simulink library "rpi_blkst"  (Simulink 7.6)
settings: Solver=ode45  StartTime=0.0  StopTime=10.0  RelTol=1e-3
settings Model: Creator=jacques  LastModifiedBy=jacques

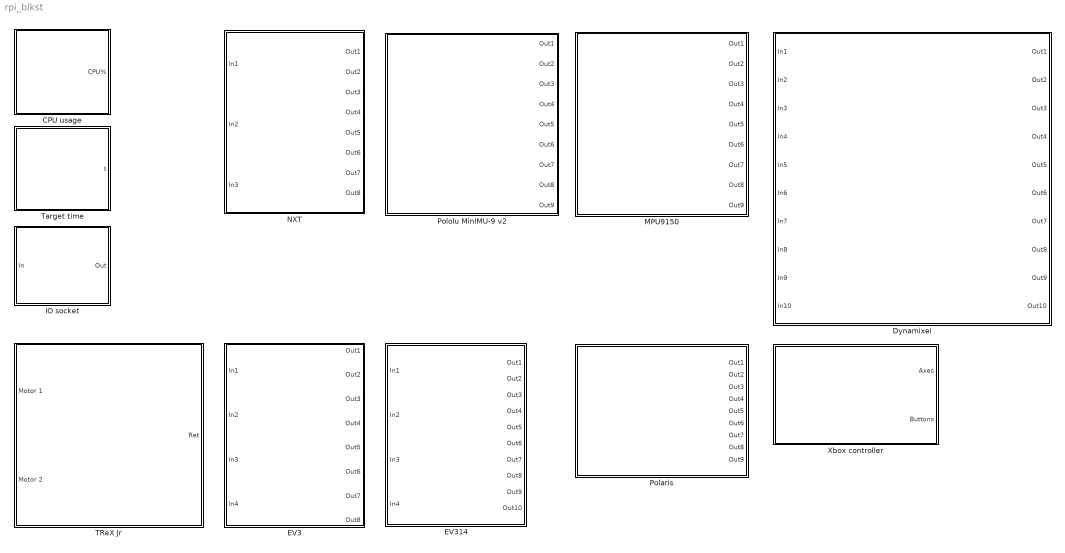
== system rpi_blkst ==
  CPU usage : Subsystem  mask(Target CPU usage){rpi_mask_Ts=0.01}
      mask prompts: rpi_mask_Ts "Sampling interval (s)"
      mask help: Percentage of CPU usage on the target. To be safe, keep below 80%.
      mask Help: Time spent in the system computation with respect to the period duration.
      mask Display: image(imread('cpu_usage.jpg'))
  Dynamixel : Subsystem  mask(Dynamixel actuator){rpi_mask_Ts=0.005, rpi_mask_portname=0, rpi_mask_baudrate=1000000, rpi_mask_startid=1, rpi_mask_nbid=1, rpi_mask_proto=2, rpi_mask_write_addr=0, rpi_mask_write_length=0, rpi_mask_read_addr=0, rpi_mask_read_length=0, rpi_mask_read_sign=0, rpi_mask_init1_addr=0, rpi_mask_init1_length=0, rpi_mask_init1_data=0, rpi_mask_init2_addr=0, rpi_mask_init2_length=0, rpi_mask_init2_data=0, rpi_mask_init3_addr=0, rpi_mask_init3_length=0, rpi_mask_init3_data=0, rpi_mask_init4_addr=0, rpi_mask_init4_length=0, rpi_mask_init4_data=0, rpi_mask_init5_addr=0, rpi_mask_init5_length=0, rpi_mask_init5_data=0, rpi_mask_init6_addr=0, rpi_mask_init6_length=0, rpi_mask_init6_data=0, rpi_mask_init7_addr=0, rpi_mask_init7_length=0, rpi_mask_init7_data=0, rpi_mask_init8_addr=0, rpi_mask_init8_length=0, rpi_mask_init8_data=0, rpi_mask_halt1_addr=0, rpi_mask_halt1_length=0, rpi_mask_halt1_data=0, rpi_mask_halt2_addr=0, rpi_mask_halt2_length=0, rpi_mask_halt2_data=0}
      mask prompts: rpi_mask_Ts "Sampling interval (s)"; rpi_mask_portname "Serial port number"; rpi_mask_baudrate "Baud rate (bps)"; rpi_mask_startid "ID of the first device"; rpi_mask_nbid "Number of devices"; rpi_mask_proto "Protocol version"; rpi_mask_write_addr "Input write address"; rpi_mask_write_length "Input write length"; rpi_mask_read_addr "Output read address"; rpi_mask_read_length "Output read length"; rpi_mask_read_sign "Output read sign"; rpi_mask_init1_addr "Address of instruction 1"; rpi_mask_init1_length "Length of instruction 1"; rpi_mask_init1_data "Data of instruction 1"; rpi_mask_init2_addr "Address of instruction 2"; rpi_mask_init2_length "Length of instruction 2"; rpi_mask_init2_data "Data of instruction 2"; rpi_mask_init3_addr "Address of instruction 3"; rpi_mask_init3_length "Length of instruction 3"; rpi_mask_init3_data "Data of instruction 3"; rpi_mask_init4_addr "Address of instruction 4"; rpi_mask_init4_length "Length of instruction 4"; rpi_mask_init4_data "Data of instruction 4"; rpi_mask_init5_addr "Address of instruction 5"; rpi_mask_init5_length "Length of instruction 5"; rpi_mask_init5_data "Data of instruction 5"; rpi_mask_init6_addr "Address of instruction 6"; rpi_mask_init6_length "Length of instruction 6"; rpi_mask_init6_data "Data of instruction 6"; rpi_mask_init7_addr "Address of instruction 7"; rpi_mask_init7_length "Length of instruction 7"; rpi_mask_init7_data "Data of instruction 7"; rpi_mask_init8_addr "Address of instruction 8"; rpi_mask_init8_length "Length of instruction 8"; rpi_mask_init8_data "Data of instruction 8"; rpi_mask_halt1_addr "Address of instruction 1"; rpi_mask_halt1_length "Length of instruction 1"; rpi_mask_halt1_data "Data of instruction 1"; rpi_mask_halt2_addr "Address of instruction 2"; rpi_mask_halt2_length "Length of instruction 2"; rpi_mask_halt2_data "Data of instruction 2"
      mask help: Control all Dynamixel actuators with Simulink coder.
      mask Help:
      | Sampling interval: should be greater than 5ms.
      | Portname: 0-9:/dev/ttyUSB0-/dev/ttyUSB9, 10-19:/dev/ttyS0-/dev/ttyS9.
      | Baudrate: the speed of the serial communication (ex: 57600).
      | StartID: the ID of the first device that should be accessed.
      | NBID: number of devices that should be addressed by this block (max 10).
      | Protocol: version of the communication protocol (1 or 2).
      | Input write address: register address where block input is written. If 0, no write is issued.
      | Input write length: dimension of the write register (1, 2 or 4 bytes).
      | Output read address: register from where the block output is read.
      | Output read length: dimension of the read register (1, 2 or 4 bytes).
      | Output read sign: 0 for an unsigned int and 1 for a signed int.
      | 
      | Tabs "Initialization" and "Shutdown" can be used to program startup and shutdown instructions.
      | 
      | Instruction address: address of the register.
      | Instruction length: size of the register (1, 2 or 4 bytes).
      | Instruction data: data written to the register.
      | If no initialization or shutdown instructions have to be sent, leave "0" as address.
      | 
      | This block can be instancied many times, even with the same port address.
      | 
      | See https://github.com/jacqu/dxl for more informations.
      mask TabNameString: General,General,General,General,General,General,I/O,I/O,I/O,I/O,I/O,Initialization,Initialization,Initialization,Initialization,Initialization,Initialization,Initialization,Initialization,Initialization,Initialization,Initialization,Initialization,Initialization,Initialization,Initialization,Initialization,Initialization,Initialization,Initialization,Initialization,Initialization,Initialization,Initialization,Initialization,Shutdown,Shutdown,Shutdown,Shutdown,Shutdown,Shutdown
      mask Display:
      | image(imread('dynamixel.jpg'))
      | port_label('input',1,'u1')
      | port_label('input',2,'u2')
      | port_label('input',3,'u3')
      | port_label('input',4,'u4')
      | port_label('input',5,'u5')
      | port_label('input',6,'u6')
      | port_label('input',7,'u7')
      | port_label('input',8,'u8')
      | port_label('input',9,'u9')
      | port_label('input',10,'u10')
      | port_label('output',1,'y1')
      | port_label('output',2,'y2')
      | port_label('output',3,'y3')
      | port_label('output',4,'y4')
      | port_label('output',5,'y5')
      | port_label('output',6,'y6')
      | port_label('output',7,'y7')
      | port_label('output',8,'y8')
      | port_label('output',9,'y9')
      | port_label('output',10,'y10')
  EV3 : Subsystem  mask(LEGO EV3){rpi_mask_Ts=0.01}
      mask prompts: rpi_mask_Ts "Sampling interval (s)"
      mask help: LEGO EV3 communication block.
      mask Help: Communicates through USB with the Lego EV3 virtual machine.
      mask Display:
      | image(imread('ev3.jpg'))
      | port_label('input',1,'A')
      | port_label('input',2,'B')
      | port_label('input',3,'C')
      | port_label('input',4,'D')
      | port_label('output',1,'A')
      | port_label('output',2,'B')
      | port_label('output',3,'C')
      | port_label('output',4,'D')
      | port_label('output',5,'1')
      | port_label('output',6,'2')
      | port_label('output',7,'3')
      | port_label('output',8,'4')
  EV314 : Subsystem  mask(EV3.14 interface){rpi_mask_ID=0, rpi_mask_Ts=0.01}
      mask prompts: rpi_mask_ID "EV3.14 block ID"; rpi_mask_Ts "Sampling interval (s)"
      mask help: Controlling an EV3 running the EV3.14 firmware through USB.
      mask Help:
      | UA, UB, UC, UD are the motor voltage control signals ranging from -10000 to +10000.
      | 
      | EA, EB, EC, ED are the encoder values. EV3.14 counts in quad-precision. Thus there is 720 increments per turn.
      | 
      | S1, S2, S3, S4 are the voltage measured at the sensor inputs. Only analog sensors are supported.
      | 
      | IBAT gives the battery current in mA.
      | 
      | VBAT gives the battery voltage in mV. Note that the brick automatically halts under 5.4V.
      | 
      | ID is the identifier of the brick. The bricks are sorted in an ascending order of hardware ID. The first ID in the list in 0.
      | 
      | The USB roundtrip transaction between the host (the target of Simulink) and the EV3 lasts 1ms.
      mask Display:
      | image(imread('ev3.14.jpg'))
      | port_label('input',1,'UA')
      | port_label('input',2,'UB')
      | port_label('input',3,'UC')
      | port_label('input',4,'UD')
      | port_label('output',1,'EA')
      | port_label('output',2,'EB')
      | port_label('output',3,'EC')
      | port_label('output',4,'ED')
      | port_label('output',5,'S1')
      | port_label('output',6,'S2')
      | port_label('output',7,'S3')
      | port_label('output',8,'S4')
      | port_label('output',9,'IBAT')
      | port_label('output',10,'VBAT')
  IO socket : Subsystem  mask(IO socket){rpi_mask_Ts=0.01, rpi_mask_ip1=127, rpi_mask_ip2=0, rpi_mask_ip3=0, rpi_mask_ip4=1}
      mask prompts: rpi_mask_Ts "Sampling interval (s)"; rpi_mask_ip1 "IP1"; rpi_mask_ip2 "IP2"; rpi_mask_ip3 "IP3"; rpi_mask_ip4 "IP4"
      mask help: Input / Output socket
      mask Help:
      | Enables a bidirectional communication with other machines using UDP sockets.
      | 
      | IP adress of the server is IP1.IP2.IP3.IP4.
      | 
      | Multiple IO socket blocks (max 10) can be used simultaneously with different IP addresses.
      | 
      | An example of server code can be found in "res/rpit_socket_server.c".
      | 
      | Minimum sampling period is 1ms.
      mask Display: image(imread('socket2.jpg'))
  MPU9150 : Subsystem  mask(MPU9150 IMU){rpi_mask_Ts=0.01}
      mask prompts: rpi_mask_Ts "Sampling interval (s)"
      mask help: Inertial Measurement Unit based on Invensense's MPU 9150 chip.
      mask Help:
      | Interface to the DroTek (www.drotek.fr), Accelerometer, and Compass board.
      | It should also work with the MPU9150 SparkFun board.
      | It is connected to the RPI through the I2C port.
      | The accelerometer and the gyro are refreshed internally at 1kHz.
      | The range of the accelerometer is +/-2g.
      | The range of the gyro is +/-1000deg/s.
      | The magnetometer is refreshed every 4 samples. It is internally refreshed at 100Hz.
      mask Display:
      | image(imread('9150.jpg'))
      | port_label('output',1,'ax')
      | port_label('output',2,'ay')
      | port_label('output',3,'az')
      | port_label('output',4,'gx')
      | port_label('output',5,'gy')
      | port_label('output',6,'gz')
      | port_label('output',7,'mx')
      | port_label('output',8,'my')
      | port_label('output',9,'mz')
  NXT : Subsystem  mask(LEGO NXT){rpi_mask_Ts=0.01, rpi_mask_id=1}
      mask prompts: rpi_mask_Ts "Sampling interval (s)"; rpi_mask_id "NXT id"
      mask help: LEGO NXT communication block.
      mask Help:
      | Communicates through USB with the Lego NXT driver.
      | The driver must be launched on the NXT.
      | Drivers are available in the "res" directory.
      | One of these NXTOSEK ".rxe" files must be downloaded to the NXT.
      | The suffix of the filename defines the id of the NXT.
      | The round-trip exchange duration between the RPI and the NXT is approx. 1ms.
      mask Display:
      | image(imread('nxt.jpg'))
      | port_label('input',1,'A')
      | port_label('input',2,'B')
      | port_label('input',3,'C')
      | port_label('output',1,'A')
      | port_label('output',2,'B')
      | port_label('output',3,'C')
      | port_label('output',4,'1')
      | port_label('output',5,'2')
      | port_label('output',6,'3')
      | port_label('output',7,'4')
      | port_label('output',8,'BAT')
  Polaris : Subsystem  mask(NDI Polaris){rpi_mask_Ts=0.01}
      mask prompts: rpi_mask_Ts "Sampling interval (s)"
      mask help:
      | Interface for the Polaris system from NDI.
      | Compatible with the original model.
      | Newer VICRA and SPECTRA are not compatible.
      mask Help:
      | The Polaris schould be connected by a serial link to the target.
      | The default serial port is /dev/ttyUSB0. It can be changed in "polaris.h".
      | 
      | The rom file should be named "polaris.rom" and put into the "blocks" directory.
      | 
      | Polaris position data are internally refreshed at 60Hz.
      | The target reads asynchronously the position.
      | So, if your discrete sampling interval is less than 16ms, expect some identical
      | frame reads.
      | 
      | Minimum sampling interval is 1ms.
      mask Display:
      | image(imread('polaris.jpg'))
      | port_label( 'output', 1, 'x' )
      | port_label( 'output', 2, 'y' )
      | port_label( 'output', 3, 'z' )
      | port_label( 'output', 4, 'q0' )
      | port_label( 'output', 5, 'qx' )
      | port_label( 'output', 6, 'qy' )
      | port_label( 'output', 7, 'qz' )
      | port_label( 'output', 8, 'state' )
      | port_label( 'output', 9, 'frame' )
  Pololu MinIMU-9 v2 : Subsystem  mask(IMU){rpi_mask_Ts=0.01}
      mask prompts: rpi_mask_Ts "Sampling interval (s)"
      mask help: Inertiel Measurement Unit
      mask Help:
      | Interface to the Pololu MinIMU-9 v2 Gyro, Accelerometer, and Compass board.
      | It is connected to the RPI through the I2C port.
      | The accelerometer is refreshed internally at 400Hz. Its range is +/-2g.
      | The gyro is refreshed at 760Hz, with a bandpass filter from 0.09Hz to 100Hz. Its range is +/-500deg/s.
      | The magnetometer is refreshed at 220Hz. Its range is +/-1.3 Gauss.
      mask Display:
      | image(imread('pololu_imu.jpg'))
      | port_label('output',1,'ax')
      | port_label('output',2,'ay')
      | port_label('output',3,'az')
      | port_label('output',4,'gx')
      | port_label('output',5,'gy')
      | port_label('output',6,'gz')
      | port_label('output',7,'mx')
      | port_label('output',8,'my')
      | port_label('output',9,'mz')
  TReX Jr : Subsystem  mask(TReX Jr){rpi_mask_trex_port=0, rpi_mask_trex_id=0, rpi_mask_Ts=0.01}
      mask prompts: rpi_mask_trex_port "Port"; rpi_mask_trex_id "ID"; rpi_mask_Ts "Sampling interval (s)"
      mask help: Pololu TReX Jr driver block
      mask Help:
      | Port:
      | * integer < 0: /dev/ttyS[-interger-1]
      | * integer >= 0: /dev/ttyUSB[integer]
      | 
      | ID: ID of the device on a daisy chain (default = 7)
      | 
      | Sampling interval: min 0.01s
      | (100Hz max frequency due to hardware limitations)
      | 
      | Motor1 and Motor2:
      | * Duty cycles for motor 1 and 2 ranging from -127 to 127
      mask Display:
      | image(imread('trex.jpg'))
      | port_label('input',1, 'M1')
      | port_label('input',2, 'M2')
      | port_label('output',1, 'Ret')
  Target time : Subsystem  mask(RPI time){rpi_mask_Ts=0.01}
      mask prompts: rpi_mask_Ts "Sampling interval (s)"
      mask help: Read absolute time on the RPI
      mask Help: Output given in seconds
      mask Display: image(imread('rtc.jpg'))
  Xbox controller : Subsystem  mask(Xbox controller){rpi_mask_ID=0, rpi_mask_Ts=0.01}
      mask prompts: rpi_mask_ID "Joystick device ID"; rpi_mask_Ts "Sampling interval (s)"
      mask help: RPIt Xbox controller
      mask Help:
      | Interfacing a Xbox controller with RPIt.
      | Works with xpad Linux driver.
      | Should work with controllers from other manufacturers.
      | This block handles 8 axes and 11 buttons.
      | Device ID: 0->/dev/input/js0, 1->/dev/input/js1,...
      | Up to 5 controllers can be used simultaneously.
      mask Display:
      | image(imread('xbox_controller.jpg'))
      | port_label('output',1,'Axes')
      | port_label('output',2,'But.')

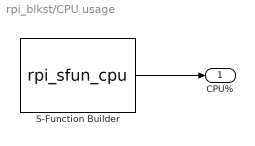
== system rpi_blkst/CPU usage ==
  S-Function Builder : S-Function  InitFcn=try, set_param(gcb,'FunctionName','rpi_sfun_cpu'), end  FunctionName=rpi_sfun_cpu  Parameters=rpi_mask_Ts  SFunctionModules=rpi_sfun_cpu_wrapper  WizardData=DataTag0  EnableBusSupport=off  mask(S-Function Builder){}
      mask help: The S-Function Builder block creates a wrapper C-MEX S-function from your supplied C code with multiple input ports, output ports, and a variable number of scalar, vector, or matrix parameters. The input and output ports can propagate Simulink built-in data types, fixed-point datatypes, complex, frame, 1-D, and 2-D signals. This block also supports discrete and continuous states of type real. You can optionally have the block generate a TLC file to be used with Real-Time Workshop for code generation.
      mask init:
      | val = [[.9  0.75 0.75 1 1 .9 .9 1]',[1 1 0.75 0.75 .9 .9 1 .9]'];try , sys = get_param(gcb,'SfunBuilderFcnName');if isempty(sys), sys = get_param(gcb,'FunctionName'); end,catch, sys = get_param(gcb,'FunctionName'); end
      settings: PreSaveFcn=try, set_param(gcb,'FunctionName','rpi_sfun_cpu'), end  OpenFcn=sfunctionwizard(gcbh)
      mask Display: plot(val(:,1),val(:,2)),disp(sys), port_label('output',1,'y0')
  CPU% : Outport
  wires:
  S-Function Builder/1 -> CPU%/1

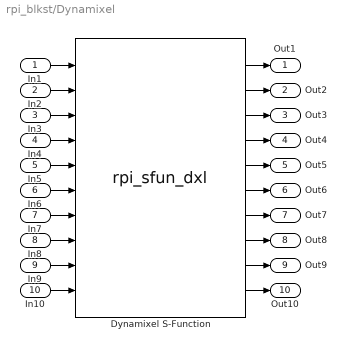
== system rpi_blkst/Dynamixel ==
  In1 : Inport
  In2 : Inport  Port=2
  In3 : Inport  Port=3
  In4 : Inport  Port=4
  In5 : Inport  Port=5
  In6 : Inport  Port=6
  In7 : Inport  Port=7
  In8 : Inport  Port=8
  In9 : Inport  Port=9
  In10 : Inport  Port=10
  Dynamixel S-Function : S-Function  InitFcn=try, set_param(gcb,'FunctionName','rpi_sfun_dxl'), end  FunctionName=rpi_sfun_dxl  Parameters=rpi_mask_Ts,uint8(rpi_mask_portname),uint32(rpi_mask_baudrate),uint8(rpi_mask_startid),uint8(rpi_mask_nbid),uint8(rpi_mask_proto),uint16(rpi_mask_write_addr),uint8(rpi_mask_write_length),uint16(rpi_mask_read_addr),uint8(rpi_mask_read_length),uint8(rpi_mask_read_sign),uint16(rpi_mask_init1_addr),uint8(rpi_mask_init1_length),rpi_mask_init1_data,uint16(rpi_mask_init2_addr),uint8(rpi_mask_init2_length),rpi_mask_init2_data,uint16(rpi_mask_init3_addr),uint8(rpi_mask_init3_length),rpi_mask_init3_data,uint16(rpi_mask_init4_addr),uint8(rpi_mask_init4_length),rpi_mask_init4_data,uint16(rpi_mask_init5_addr),uint8(rpi_mask_init5_length),rpi_mask_init5_data,uint16(rpi_mask_init6_addr),uint8(rpi_mask_init6_length),rpi_mask_init6_data,uint16(rpi_mask_init7_addr),uint8(rpi_mask_init7_length),rpi_mask_init7_data,uint16(rpi_mask_init8_addr),uint8(rpi_mask_init8_length),rpi_mask_init8_data,uint16(rpi_mask_halt1_addr),uint8(rpi_mask_halt1_length),rpi_mask_halt1_data,uint16(rpi_mask_halt2_addr),uint8(rpi_mask_halt2_length),rpi_mask_halt2_data  SFunctionModules=rpi_sfun_dxl_wrapper  WizardData=DataTag1  EnableBusSupport=off  mask(S-Function Builder){}
      mask help: The S-Function Builder block creates a wrapper C-MEX S-function from your supplied C code with multiple input ports, output ports, and a variable number of scalar, vector, or matrix parameters. The input and output ports can propagate Simulink built-in data types, fixed-point datatypes, complex, frame, 1-D, and 2-D signals. This block also supports discrete and continuous states of type real. You can optionally have the block generate a TLC file to be used with Real-Time Workshop for code generation.
      mask init: same as rpi_blkst/CPU usage/S-Function Builder
      settings: PreSaveFcn=try, set_param(gcb,'FunctionName','rpi_sfun_dxl'), end  OpenFcn=sfunctionwizard(gcbh)
      mask Display: plot(val(:,1),val(:,2)),disp(sys), port_label('input',1,'u1'), port_label('input',2,'u2'), port_label('input',3,'u3'), port_label('input',4,'u4'), port_label('input',5,'u5'), port_label('input',6,'u6'), port_label('input',7,'u7'), port_label('input',8,'u8'), port_label('input',9,'u9'), port_label('input',10,'u10'), port_label('output',1,'y1'), port_label('output',2,'y2'), port_label('output',3,'y3'), port_label('output',4,'y4'), port_label('output',5,'y5'), port_label('output',6,'y6'), port_label('output',7,'y7'), port_label('output',8,'y8'), port_label('output',9,'y9'), port_label('output',10,'y10')
  Out1 : Outport
  Out2 : Outport  Port=2
  Out3 : Outport  Port=3
  Out4 : Outport  Port=4
  Out5 : Outport  Port=5
  Out6 : Outport  Port=6
  Out7 : Outport  Port=7
  Out8 : Outport  Port=8
  Out9 : Outport  Port=9
  Out10 : Outport  Port=10
  wires:
  In1/1 -> Dynamixel S-Function/1
  Dynamixel S-Function/1 -> Out1/1
  In2/1 -> Dynamixel S-Function/2
  Dynamixel S-Function/2 -> Out2/1
  In3/1 -> Dynamixel S-Function/3
  Dynamixel S-Function/3 -> Out3/1
  In4/1 -> Dynamixel S-Function/4
  Dynamixel S-Function/4 -> Out4/1
  In5/1 -> Dynamixel S-Function/5
  Dynamixel S-Function/5 -> Out5/1
  In6/1 -> Dynamixel S-Function/6
  Dynamixel S-Function/6 -> Out6/1
  In7/1 -> Dynamixel S-Function/7
  Dynamixel S-Function/7 -> Out7/1
  In8/1 -> Dynamixel S-Function/8
  Dynamixel S-Function/8 -> Out8/1
  In9/1 -> Dynamixel S-Function/9
  Dynamixel S-Function/9 -> Out9/1
  In10/1 -> Dynamixel S-Function/10
  Dynamixel S-Function/10 -> Out10/1

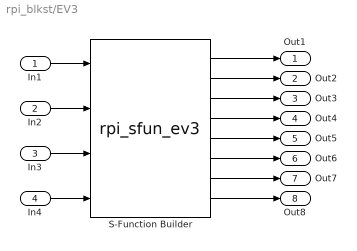
== system rpi_blkst/EV3 ==
  In1 : Inport
  In2 : Inport  Port=2
  In3 : Inport  Port=3
  In4 : Inport  Port=4
  S-Function Builder : S-Function  InitFcn=try, set_param(gcb,'FunctionName','rpi_sfun_ev3'), end  FunctionName=rpi_sfun_ev3  Parameters=rpi_mask_Ts  SFunctionModules=rpi_sfun_ev3_wrapper  WizardData=DataTag2  EnableBusSupport=off  mask(S-Function Builder){}
      mask help: The S-Function Builder block creates a wrapper C-MEX S-function from your supplied C code with multiple input ports, output ports, and a variable number of scalar, vector, or matrix parameters. The input and output ports can propagate Simulink built-in data types, fixed-point datatypes, complex, frame, 1-D, and 2-D signals. This block also supports discrete and continuous states of type real. You can optionally have the block generate a TLC file to be used with Real-Time Workshop for code generation.
      mask init: same as rpi_blkst/CPU usage/S-Function Builder
      settings: PreSaveFcn=try, set_param(gcb,'FunctionName','rpi_sfun_ev3'), end  OpenFcn=sfunctionwizard(gcbh)
      mask Display: plot(val(:,1),val(:,2)),disp(sys), port_label('input',1,'u_A'), port_label('input',2,'u_B'), port_label('input',3,'u_C'), port_label('input',4,'u_D'), port_label('output',1,'y_A'), port_label('output',2,'y_B'), port_label('output',3,'y_C'), port_label('output',4,'y_D'), port_label('output',5,'y_1'), port_label('output',6,'y_2'), port_label('output',7,'y_3'), port_label('output',8,'y_4')
  Out1 : Outport
  Out2 : Outport  Port=2
  Out3 : Outport  Port=3
  Out4 : Outport  Port=4
  Out5 : Outport  Port=5
  Out6 : Outport  Port=6
  Out7 : Outport  Port=7
  Out8 : Outport  Port=8
  wires:
  In1/1 -> S-Function Builder/1
  In2/1 -> S-Function Builder/2
  In3/1 -> S-Function Builder/3
  In4/1 -> S-Function Builder/4
  S-Function Builder/1 -> Out1/1
  S-Function Builder/2 -> Out2/1
  S-Function Builder/3 -> Out3/1
  S-Function Builder/4 -> Out4/1
  S-Function Builder/5 -> Out5/1
  S-Function Builder/6 -> Out6/1
  S-Function Builder/7 -> Out7/1
  S-Function Builder/8 -> Out8/1

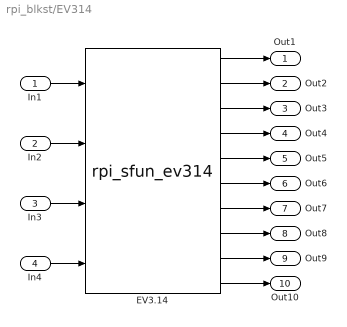
== system rpi_blkst/EV314 ==
  In1 : Inport
  In2 : Inport  Port=2
  In3 : Inport  Port=3
  In4 : Inport  Port=4
  EV3.14 : S-Function  InitFcn=try, set_param(gcb,'FunctionName','rpi_sfun_ev314'), end  FunctionName=rpi_sfun_ev314  Parameters=rpi_mask_Ts,uint8(rpi_mask_ID)  SFunctionModules=rpi_sfun_ev314_wrapper  WizardData=DataTag3  EnableBusSupport=off  mask(S-Function Builder){}
      mask help: The S-Function Builder block creates a wrapper C-MEX S-function from your supplied C code with multiple input ports, output ports, and a variable number of scalar, vector, or matrix parameters. The input and output ports can propagate Simulink built-in data types, fixed-point datatypes, complex, frame, 1-D, and 2-D signals. This block also supports discrete and continuous states of type real. You can optionally have the block generate a TLC file to be used with Real-Time Workshop for code generation.
      mask init: same as rpi_blkst/CPU usage/S-Function Builder
      settings: PreSaveFcn=try, set_param(gcb,'FunctionName','rpi_sfun_ev314'), end  OpenFcn=sfunctionwizard(gcbh)
      mask Display: plot(val(:,1),val(:,2)),disp(sys), port_label('input',1,'UA'), port_label('input',2,'UB'), port_label('input',3,'UC'), port_label('input',4,'UD'), port_label('output',1,'EA'), port_label('output',2,'EB'), port_label('output',3,'EC'), port_label('output',4,'ED'), port_label('output',5,'S1'), port_label('output',6,'S2'), port_label('output',7,'S3'), port_label('output',8,'S4'), port_label('output',9,'IBAT'), port_label('output',10,'VBAT')
  Out1 : Outport
  Out2 : Outport  Port=2
  Out3 : Outport  Port=3
  Out4 : Outport  Port=4
  Out5 : Outport  Port=5
  Out6 : Outport  Port=6
  Out7 : Outport  Port=7
  Out8 : Outport  Port=8
  Out9 : Outport  Port=9
  Out10 : Outport  Port=10
  wires:
  In1/1 -> EV3.14/1
  In2/1 -> EV3.14/2
  In3/1 -> EV3.14/3
  In4/1 -> EV3.14/4
  EV3.14/1 -> Out1/1
  EV3.14/2 -> Out2/1
  EV3.14/3 -> Out3/1
  EV3.14/4 -> Out4/1
  EV3.14/5 -> Out5/1
  EV3.14/6 -> Out6/1
  EV3.14/7 -> Out7/1
  EV3.14/8 -> Out8/1
  EV3.14/9 -> Out9/1
  EV3.14/10 -> Out10/1

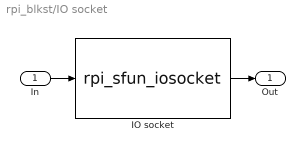
== system rpi_blkst/IO socket ==
  In : Inport
  IO socket : S-Function  InitFcn=try, set_param(gcb,'FunctionName','rpi_sfun_iosocket'), end  FunctionName=rpi_sfun_iosocket  Parameters=rpi_mask_Ts,uint8(rpi_mask_ip1),uint8(rpi_mask_ip2),uint8(rpi_mask_ip3),uint8(rpi_mask_ip4)  SFunctionModules=rpi_sfun_iosocket_wrapper  WizardData=DataTag4  EnableBusSupport=off  mask(S-Function Builder){}
      mask help: The S-Function Builder block creates a wrapper C-MEX S-function from your supplied C code with multiple input ports, output ports, and a variable number of scalar, vector, or matrix parameters. The input and output ports can propagate Simulink built-in data types, fixed-point datatypes, complex, frame, 1-D, and 2-D signals. This block also supports discrete and continuous states of type real. You can optionally have the block generate a TLC file to be used with Real-Time Workshop for code generation.
      mask init: same as rpi_blkst/CPU usage/S-Function Builder
      settings: PreSaveFcn=try, set_param(gcb,'FunctionName','rpi_sfun_iosocket'), end  OpenFcn=sfunctionwizard(gcbh)
      mask Display: plot(val(:,1),val(:,2)),disp(sys), port_label('input',1,'u0'), port_label('output',1,'y0')
  Out : Outport
  wires:
  In/1 -> IO socket/1
  IO socket/1 -> Out/1

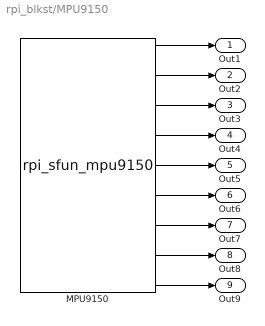
== system rpi_blkst/MPU9150 ==
  MPU9150 : S-Function  InitFcn=try, set_param(gcb,'FunctionName','rpi_sfun_mpu9150'), end  FunctionName=rpi_sfun_mpu9150  Parameters=rpi_mask_Ts  SFunctionModules=rpi_sfun_mpu9150_wrapper  WizardData=DataTag5  EnableBusSupport=off  mask(S-Function Builder){}
      mask help: The S-Function Builder block creates a wrapper C-MEX S-function from your supplied C code with multiple input ports, output ports, and a variable number of scalar, vector, or matrix parameters. The input and output ports can propagate Simulink built-in data types, fixed-point datatypes, complex, frame, 1-D, and 2-D signals. This block also supports discrete and continuous states of type real. You can optionally have the block generate a TLC file to be used with Real-Time Workshop for code generation.
      mask init: same as rpi_blkst/CPU usage/S-Function Builder
      settings: PreSaveFcn=try, set_param(gcb,'FunctionName','rpi_sfun_mpu9150'), end  OpenFcn=sfunctionwizard(gcbh)
      mask Display: plot(val(:,1),val(:,2)),disp(sys), port_label('output',1,'ax'), port_label('output',2,'ay'), port_label('output',3,'az'), port_label('output',4,'gx'), port_label('output',5,'gy'), port_label('output',6,'gz'), port_label('output',7,'mx'), port_label('output',8,'my'), port_label('output',9,'mz')
  Out1 : Outport
  Out2 : Outport  Port=2
  Out3 : Outport  Port=3
  Out4 : Outport  Port=4
  Out5 : Outport  Port=5
  Out6 : Outport  Port=6
  Out7 : Outport  Port=7
  Out8 : Outport  Port=8
  Out9 : Outport  Port=9
  wires:
  MPU9150/1 -> Out1/1
  MPU9150/2 -> Out2/1
  MPU9150/3 -> Out3/1
  MPU9150/4 -> Out4/1
  MPU9150/5 -> Out5/1
  MPU9150/6 -> Out6/1
  MPU9150/7 -> Out7/1
  MPU9150/8 -> Out8/1
  MPU9150/9 -> Out9/1

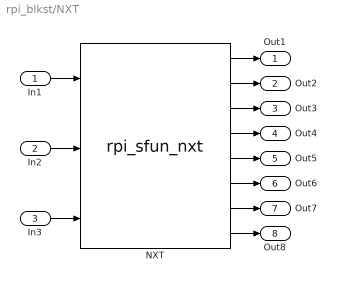
== system rpi_blkst/NXT ==
  In1 : Inport
  In2 : Inport  Port=2
  In3 : Inport  Port=3
  NXT : S-Function  InitFcn=try, set_param(gcb,'FunctionName','rpi_sfun_nxt'), end  FunctionName=rpi_sfun_nxt  Parameters=rpi_mask_Ts,uint32(rpi_mask_id)  SFunctionModules=rpi_sfun_nxt_wrapper  WizardData=DataTag6  EnableBusSupport=off  mask(S-Function Builder){}
      mask help: The S-Function Builder block creates a wrapper C-MEX S-function from your supplied C code with multiple input ports, output ports, and a variable number of scalar, vector, or matrix parameters. The input and output ports can propagate Simulink built-in data types, fixed-point datatypes, complex, frame, 1-D, and 2-D signals. This block also supports discrete and continuous states of type real. You can optionally have the block generate a TLC file to be used with Real-Time Workshop for code generation.
      mask init: same as rpi_blkst/CPU usage/S-Function Builder
      settings: PreSaveFcn=try, set_param(gcb,'FunctionName','rpi_sfun_nxt'), end  OpenFcn=sfunctionwizard(gcbh)
      mask Display: plot(val(:,1),val(:,2)),disp(sys), port_label('input',1,'u_A'), port_label('input',2,'u_B'), port_label('input',3,'u_C'), port_label('output',1,'y_A'), port_label('output',2,'y_B'), port_label('output',3,'y_C'), port_label('output',4,'y_1'), port_label('output',5,'y_2'), port_label('output',6,'y_3'), port_label('output',7,'y_4'), port_label('output',8,'bat')
  Out1 : Outport
  Out2 : Outport  Port=2
  Out3 : Outport  Port=3
  Out4 : Outport  Port=4
  Out5 : Outport  Port=5
  Out6 : Outport  Port=6
  Out7 : Outport  Port=7
  Out8 : Outport  Port=8
  wires:
  NXT/1 -> Out1/1
  In1/1 -> NXT/1
  NXT/2 -> Out2/1
  NXT/3 -> Out3/1
  NXT/4 -> Out4/1
  NXT/5 -> Out5/1
  NXT/6 -> Out6/1
  NXT/7 -> Out7/1
  NXT/8 -> Out8/1
  In2/1 -> NXT/2
  In3/1 -> NXT/3

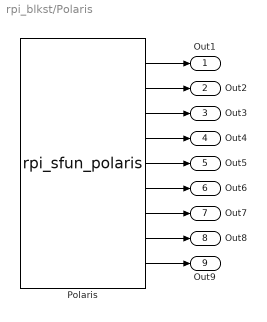
== system rpi_blkst/Polaris ==
  Polaris : S-Function  InitFcn=try, set_param(gcb,'FunctionName','rpi_sfun_polaris'), end  FunctionName=rpi_sfun_polaris  Parameters=rpi_mask_Ts  SFunctionModules=rpi_sfun_polaris_wrapper  WizardData=DataTag7  EnableBusSupport=off  mask(S-Function Builder){}
      mask help: The S-Function Builder block creates a wrapper C-MEX S-function from your supplied C code with multiple input ports, output ports, and a variable number of scalar, vector, or matrix parameters. The input and output ports can propagate Simulink built-in data types, fixed-point datatypes, complex, frame, 1-D, and 2-D signals. This block also supports discrete and continuous states of type real. You can optionally have the block generate a TLC file to be used with Real-Time Workshop for code generation.
      mask init: same as rpi_blkst/CPU usage/S-Function Builder
      settings: PreSaveFcn=try, set_param(gcb,'FunctionName','rpi_sfun_polaris'), end  OpenFcn=sfunctionwizard(gcbh)
      mask Display: plot(val(:,1),val(:,2)),disp(sys), port_label('output',1,'x'), port_label('output',2,'y'), port_label('output',3,'z'), port_label('output',4,'q0'), port_label('output',5,'qx'), port_label('output',6,'qy'), port_label('output',7,'qz'), port_label('output',8,'state'), port_label('output',9,'frame')
  Out1 : Outport
  Out2 : Outport  Port=2
  Out3 : Outport  Port=3
  Out4 : Outport  Port=4
  Out5 : Outport  Port=5
  Out6 : Outport  Port=6
  Out7 : Outport  Port=7
  Out8 : Outport  Port=8
  Out9 : Outport  Port=9
  wires:
  Polaris/1 -> Out1/1
  Polaris/2 -> Out2/1
  Polaris/3 -> Out3/1
  Polaris/4 -> Out4/1
  Polaris/5 -> Out5/1
  Polaris/6 -> Out6/1
  Polaris/7 -> Out7/1
  Polaris/8 -> Out8/1
  Polaris/9 -> Out9/1

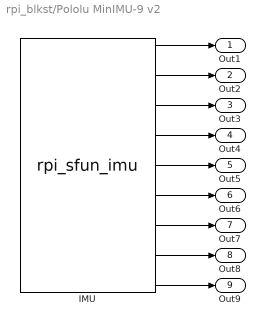
== system rpi_blkst/Pololu MinIMU-9 v2 ==
  IMU : S-Function  InitFcn=try, set_param(gcb,'FunctionName','rpi_sfun_imu'), end  FunctionName=rpi_sfun_imu  Parameters=rpi_mask_Ts  SFunctionModules=rpi_sfun_imu_wrapper  WizardData=DataTag8  EnableBusSupport=off  mask(S-Function Builder){}
      mask help: The S-Function Builder block creates a wrapper C-MEX S-function from your supplied C code with multiple input ports, output ports, and a variable number of scalar, vector, or matrix parameters. The input and output ports can propagate Simulink built-in data types, fixed-point datatypes, complex, frame, 1-D, and 2-D signals. This block also supports discrete and continuous states of type real. You can optionally have the block generate a TLC file to be used with Real-Time Workshop for code generation.
      mask init: same as rpi_blkst/CPU usage/S-Function Builder
      settings: PreSaveFcn=try, set_param(gcb,'FunctionName','rpi_sfun_imu'), end  OpenFcn=sfunctionwizard(gcbh)
      mask Display: plot(val(:,1),val(:,2)),disp(sys), port_label('output',1,'ax'), port_label('output',2,'ay'), port_label('output',3,'az'), port_label('output',4,'gx'), port_label('output',5,'gy'), port_label('output',6,'gz'), port_label('output',7,'mx'), port_label('output',8,'my'), port_label('output',9,'mz')
  Out1 : Outport
  Out2 : Outport  Port=2
  Out3 : Outport  Port=3
  Out4 : Outport  Port=4
  Out5 : Outport  Port=5
  Out6 : Outport  Port=6
  Out7 : Outport  Port=7
  Out8 : Outport  Port=8
  Out9 : Outport  Port=9
  wires:
  IMU/9 -> Out9/1
  IMU/8 -> Out8/1
  IMU/7 -> Out7/1
  IMU/6 -> Out6/1
  IMU/5 -> Out5/1
  IMU/4 -> Out4/1
  IMU/3 -> Out3/1
  IMU/2 -> Out2/1
  IMU/1 -> Out1/1

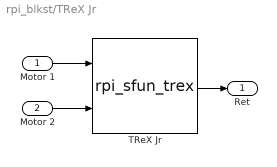
== system rpi_blkst/TReX Jr ==
  Motor 1 : Inport
  Motor 2 : Inport  Port=2
  TReX Jr : S-Function  InitFcn=try, set_param(gcb,'FunctionName','rpi_sfun_trex'), end  FunctionName=rpi_sfun_trex  Parameters=int8(rpi_mask_trex_port),uint8(rpi_mask_trex_id),rpi_mask_Ts  SFunctionModules=rpi_sfun_trex_wrapper  WizardData=DataTag9  EnableBusSupport=off  mask(S-Function Builder){}
      mask help: The S-Function Builder block creates a wrapper C-MEX S-function from your supplied C code with multiple input ports, output ports, and a variable number of scalar, vector, or matrix parameters. The input and output ports can propagate Simulink built-in data types, fixed-point datatypes, complex, frame, 1-D, and 2-D signals. This block also supports discrete and continuous states of type real. You can optionally have the block generate a TLC file to be used with Real-Time Workshop for code generation.
      mask init: same as rpi_blkst/CPU usage/S-Function Builder
      settings: CopyFcn=set_param(gcbh,'LinkStatus','none')  PreSaveFcn=try, set_param(gcb,'FunctionName','rpi_sfun_trex'), end  OpenFcn=sfunctionwizard(gcbh)
      mask Display: plot(val(:,1),val(:,2)),disp(sys), port_label('input',1,'u1'), port_label('input',2,'u2'), port_label('output',1,'Err')
  Ret : Outport
  wires:
  Motor 1/1 -> TReX Jr/1
  Motor 2/1 -> TReX Jr/2
  TReX Jr/1 -> Ret/1

== system rpi_blkst/Target time ==
  RPI time : S-Function  InitFcn=try, set_param(gcb,'FunctionName','rpi_sfun_time'), end  FunctionName=rpi_sfun_time  Parameters=rpi_mask_Ts  SFunctionModules=rpi_sfun_time_wrapper  WizardData=DataTag10  EnableBusSupport=off  mask(S-Function Builder){}
      mask help: The S-Function Builder block creates a wrapper C-MEX S-function from your supplied C code with multiple input ports, output ports, and a variable number of scalar, vector, or matrix parameters. The input and output ports can propagate Simulink built-in data types, fixed-point datatypes, complex, frame, 1-D, and 2-D signals. This block also supports discrete and continuous states of type real. You can optionally have the block generate a TLC file to be used with Real-Time Workshop for code generation.
      mask init: same as rpi_blkst/CPU usage/S-Function Builder
      settings: PreSaveFcn=try, set_param(gcb,'FunctionName','rpi_sfun_time'), end  OpenFcn=sfunctionwizard(gcbh)
      mask Display: plot(val(:,1),val(:,2)),disp(sys), port_label('output',1,'y0')
  t : Outport
  wires:
  RPI time/1 -> t/1

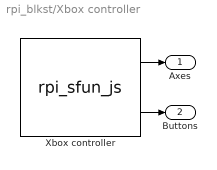
== system rpi_blkst/Xbox controller ==
  Xbox controller : S-Function  InitFcn=try, set_param(gcb,'FunctionName','rpi_sfun_js'), end  FunctionName=rpi_sfun_js  Parameters=rpi_mask_ID,rpi_mask_Ts  SFunctionModules=rpi_sfun_js_wrapper  WizardData=DataTag11  EnableBusSupport=off  mask(S-Function Builder){}
      mask help: The S-Function Builder block creates a wrapper C-MEX S-function from your supplied C code with multiple input ports, output ports, and a variable number of scalar, vector, or matrix parameters. The input and output ports can propagate Simulink built-in data types, fixed-point datatypes, complex, frame, 1-D, and 2-D signals. This block also supports discrete and continuous states of type real. You can optionally have the block generate a TLC file to be used with Real-Time Workshop for code generation.
      mask init: same as rpi_blkst/CPU usage/S-Function Builder
      settings: PreSaveFcn=try, set_param(gcb,'FunctionName','rpi_sfun_js'), end  OpenFcn=sfunctionwizard(gcbh)
      mask Display: plot(val(:,1),val(:,2)),disp(sys), port_label('output',1,'Axes'), port_label('output',2,'Buttons')
  Axes : Outport
  Buttons : Outport  Port=2
  wires:
  Xbox controller/1 -> Axes/1
  Xbox controller/2 -> Buttons/1
